simulink library "Lib_FileLogger"  (R2012b)
settings: Solver=ode45  StartTime=0.0  StopTime=10.0  RelTol=1e-3
undefined symbols (not defined in the file): macaddr, modelConstants
libraries: Lib_FileLogger x5, simulink x3, xpcethernetlib x2, xpcutilitieslib x1, dspswit3 x1, dspmtrx3 x1
settings Model: Creator=gilja  LastModifiedBy=nptl

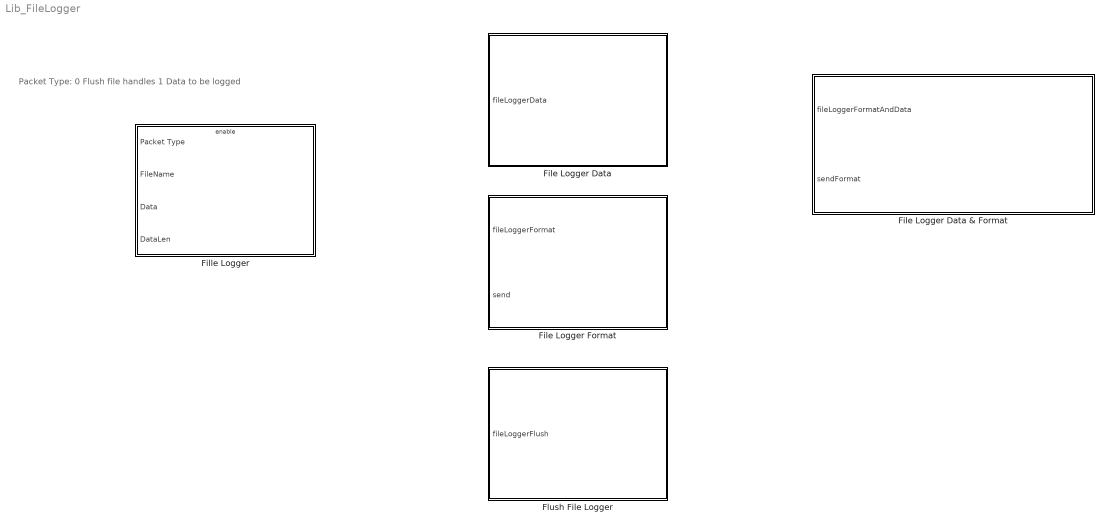
== system Lib_FileLogger ==
  note: Packet Type:
      | 0 Flush file handles
      | 1 Data to be logged
  File Logger Data : Subsystem
  File Logger Data & Format : Subsystem
  File Logger Format : Subsystem
  Fille Logger : Subsystem
  Flush File Logger : Subsystem

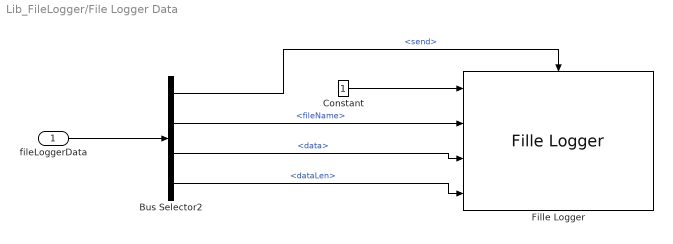
== system Lib_FileLogger/File Logger Data ==
  fileLoggerData : Inport  OutDataTypeStr=Bus: fileLoggerData
  Bus Selector2 : BusSelector  OutputSignals=send,fileName,data,dataLen
  Constant : Constant  OutDataTypeStr=boolean
  Fille Logger : Lib_FileLogger/Fille Logger
  wires:
  fileLoggerData/1 -> Bus Selector2/1
  Constant/1 -> Fille Logger/1
  Bus Selector2/1 -> Fille Logger/Enable  "<send>"
  Bus Selector2/4 -> Fille Logger/4  "<dataLen>"
  Bus Selector2/3 -> Fille Logger/3  "<data>"
  Bus Selector2/2 -> Fille Logger/2  "<fileName>"

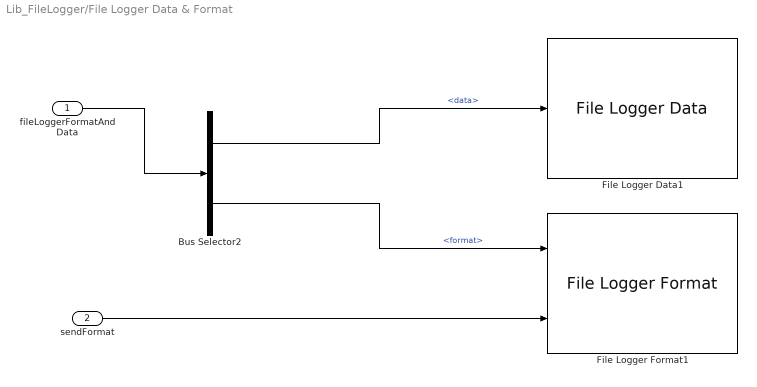
== system Lib_FileLogger/File Logger Data & Format ==
  fileLoggerFormatAndData : Inport  OutDataTypeStr=Bus: fileLoggerFormatAndData
  sendFormat : Inport  Port=2  OutDataTypeStr=boolean
  Bus Selector2 : BusSelector  OutputSignals=data,format
  File Logger Data1 : Lib_FileLogger/File Logger Data
  File Logger Format1 : Lib_FileLogger/File Logger Format
  wires:
  fileLoggerFormatAndData/1 -> Bus Selector2/1
  Bus Selector2/1 -> File Logger Data1/1  "<data>"
  Bus Selector2/2 -> File Logger Format1/1  "<format>"
  sendFormat/1 -> File Logger Format1/2

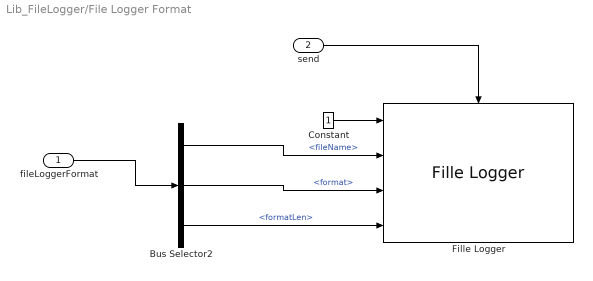
== system Lib_FileLogger/File Logger Format ==
  fileLoggerFormat : Inport  OutDataTypeStr=Bus: fileLoggerFormat
  send : Inport  Port=2  OutDataTypeStr=boolean
  Bus Selector2 : BusSelector  OutputSignals=fileName,format,formatLen
  Constant : Constant  OutDataTypeStr=boolean
  Fille Logger : Lib_FileLogger/Fille Logger
  wires:
  fileLoggerFormat/1 -> Bus Selector2/1
  send/1 -> Fille Logger/Enable
  Constant/1 -> Fille Logger/1
  Bus Selector2/3 -> Fille Logger/4  "<formatLen>"
  Bus Selector2/2 -> Fille Logger/3  "<format>"
  Bus Selector2/1 -> Fille Logger/2  "<fileName>"

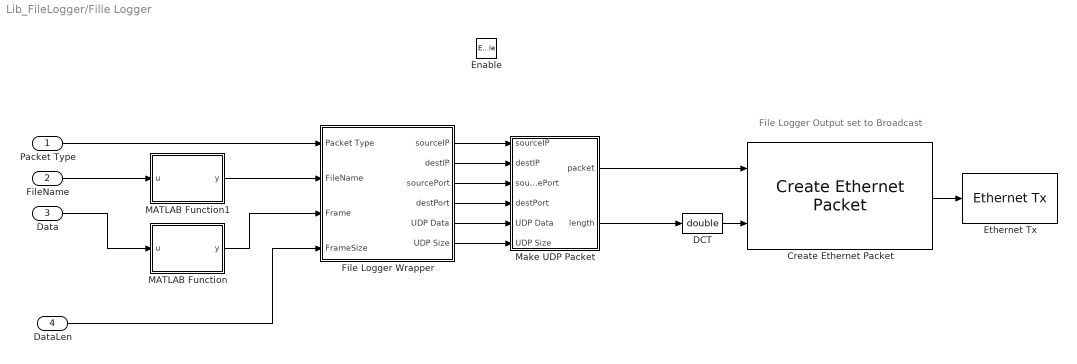
== system Lib_FileLogger/Fille Logger ==
  note: File Logger Output set to Broadcast
  Packet Type : Inport
  FileName : Inport  Port=2
  Data : Inport  Port=3
  DataLen : Inport  Port=4
  Enable : EnablePort
  "Create Ethernet Packet " : xpcethernetlib/Create Ethernet Packet   DstMac=macaddr('FF:FF:FF:FF:FF:FF')  EtherType=hex2dec('0800')
  DCT : DataTypeConversion  OutDataTypeStr=double
  "Ethernet Tx " : xpcethernetlib/Ethernet Tx   ID=2  SampleTime=-1
  File Logger Wrapper : Subsystem
  MATLAB Function : MATLAB Function  TreatAsAtomicUnit=on
  MATLAB Function1 : MATLAB Function  TreatAsAtomicUnit=on
  Make UDP Packet : Subsystem
  wires:
  FileName/1 -> MATLAB Function1/1(u)
  Data/1 -> MATLAB Function/1(u)
  File Logger Wrapper/1(sourceIP) -> Make UDP Packet/1(sourceIP)
  File Logger Wrapper/4(destPort) -> Make UDP Packet/4(destPort)
  Make UDP Packet/1(packet) -> "Create Ethernet Packet "/1
  "Create Ethernet Packet "/1 -> "Ethernet Tx "/1
  File Logger Wrapper/3(sourcePort) -> Make UDP Packet/3(sourcePort)
  Packet Type/1 -> File Logger Wrapper/1(Packet Type)
  MATLAB Function1/1(y) -> File Logger Wrapper/2(FileName)
  DCT/1 -> "Create Ethernet Packet "/2
  File Logger Wrapper/6(UDP Size) -> Make UDP Packet/6(UDP Size)
  Make UDP Packet/2(length) -> DCT/1
  DataLen/1 -> File Logger Wrapper/4(FrameSize)
  File Logger Wrapper/5(UDP Data) -> Make UDP Packet/5(UDP Data)
  File Logger Wrapper/2(destIP) -> Make UDP Packet/2(destIP)
  MATLAB Function/1(y) -> File Logger Wrapper/3(Frame)

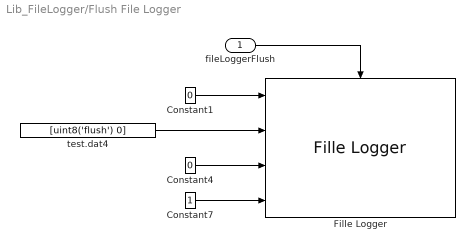
== system Lib_FileLogger/Flush File Logger ==
  fileLoggerFlush : Inport  OutDataTypeStr=boolean
  Constant1 : Constant  Value=0  OutDataTypeStr=boolean
  Constant4 : Constant  Value=0  OutDataTypeStr=boolean
  Constant7 : Constant  OutDataTypeStr=uint16
  Fille Logger : Lib_FileLogger/Fille Logger
  test.dat4 : Constant  Value=[uint8('flush') 0]  OutDataTypeStr=uint8
  wires:
  Constant4/1 -> Fille Logger/3
  fileLoggerFlush/1 -> Fille Logger/Enable
  Constant7/1 -> Fille Logger/4
  Constant1/1 -> Fille Logger/1
  test.dat4/1 -> Fille Logger/2

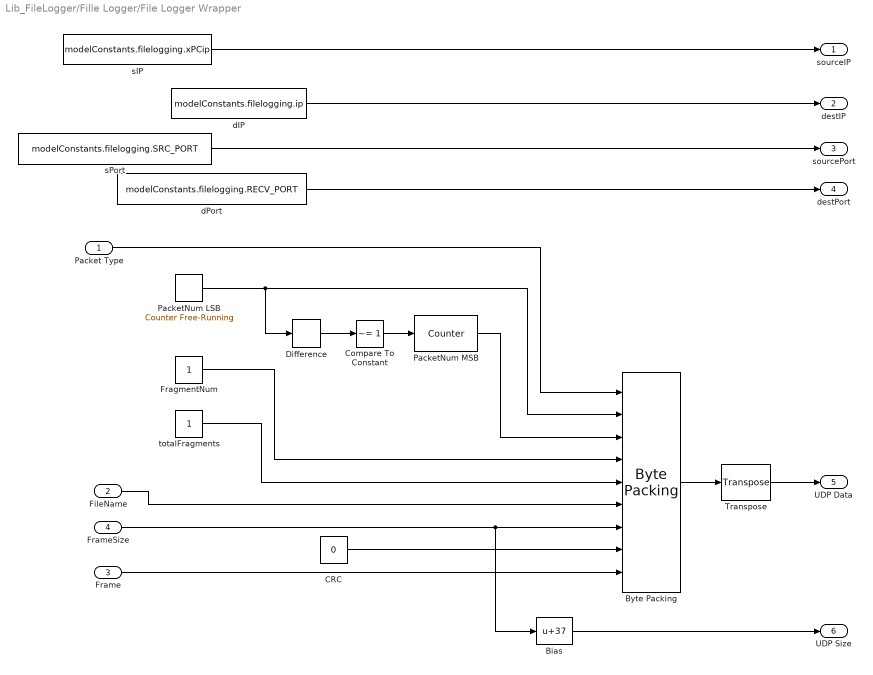
== system Lib_FileLogger/Fille Logger/File Logger Wrapper ==
  Packet Type : Inport
  FileName : Inport  Port=2
  Frame : Inport  Port=3
  FrameSize : Inport  Port=4
  Bias : Bias  Bias=37
  "Byte Packing " : xpcutilitieslib/Byte Packing   MaskPackedDataType=uint8  MaskUnpackedDataTypes={'boolean' 'uint32' 'uint32' 'uint8' 'uint8' 'uint8' 'uint16' 'uint32' 'uint8'}  MaskAlignment=1
  CRC : Constant  Value=0  OutDataTypeStr=uint32
  Compare To Constant : simulink/Logic and Bit Operations/Compare To Constant  relop=~=  const=1  OutDataTypeStr=uint8  ZeroCross=off
  Difference : simulink/Discrete/Difference  ICPrevInput=0  InputProcessing=Inherited  OutMin=[]  OutMax=[]  OutDataType=fixdt(1, 16)  OutScaling=2^-10  DoSatur=off
  FragmentNum : Constant  OutDataTypeStr=uint8
  PacketNum LSB : simulink/Sources/Counter Free-Running  NumBits=32  tsamp=-1
  PacketNum MSB : dspswit3/Counter  Direction=Up  CountEvent=Non-zero sample  CounterSize=32 bits  MaxCount=255  InitialCount=0  Output=Count  HitValue=32  ResetInput=off  SamplesPerFrame=1  Ts=1  CntDtype=uint32  HitDtype=Logical
  Transpose : dspmtrx3/Transpose  Hermitian=off  overflowFlag=off
  dIP : Constant  Value=modelConstants.filelogging.ip  OutDataTypeStr=uint8
  dPort : Constant  Value=modelConstants.filelogging.RECV_PORT  OutDataTypeStr=uint16
  sIP : Constant  Value=modelConstants.filelogging.xPCip  OutDataTypeStr=uint8
  sPort : Constant  Value=modelConstants.filelogging.SRC_PORT  OutDataTypeStr=uint16
  totalFragments : Constant  OutDataTypeStr=uint8
  sourceIP : Outport
  destIP : Outport  Port=2
  sourcePort : Outport  Port=3
  destPort : Outport  Port=4
  UDP Data : Outport  Port=5
  UDP Size : Outport  Port=6
  wires:
  Transpose/1 -> UDP Data/1
  "Byte Packing "/1 -> Transpose/1
  Frame/1 -> "Byte Packing "/9
  FrameSize/1 -> Bias/1, "Byte Packing "/7
  CRC/1 -> "Byte Packing "/8
  PacketNum MSB/1 -> "Byte Packing "/3
  Compare To Constant/1 -> PacketNum MSB/1
  Difference/1 -> Compare To Constant/1
  Packet Type/1 -> "Byte Packing "/1
  PacketNum LSB/1 -> "Byte Packing "/2, Difference/1
  FragmentNum/1 -> "Byte Packing "/4
  totalFragments/1 -> "Byte Packing "/5
  FileName/1 -> "Byte Packing "/6
  Bias/1 -> UDP Size/1
  dPort/1 -> destPort/1
  sPort/1 -> sourcePort/1
  dIP/1 -> destIP/1
  sIP/1 -> sourceIP/1

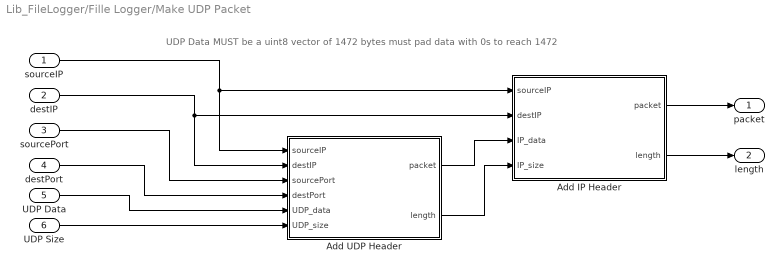
== system Lib_FileLogger/Fille Logger/Make UDP Packet ==
  note: UDP Data MUST be a uint8 vector of 1472 bytes
      | must pad data with 0s to reach 1472
  sourceIP : Inport
  destIP : Inport  Port=2
  sourcePort : Inport  Port=3
  destPort : Inport  Port=4
  UDP Data : Inport  Port=5
  UDP Size : Inport  Port=6
  Add IP Header : MATLAB Function  TreatAsAtomicUnit=on
  Add UDP Header : MATLAB Function  TreatAsAtomicUnit=on
  packet : Outport
  length : Outport  Port=2
  wires:
  UDP Size/1 -> Add UDP Header/6(UDP_size)
  Add IP Header/2(length) -> length/1
  Add IP Header/1(packet) -> packet/1
  UDP Data/1 -> Add UDP Header/5(UDP_data)
  destPort/1 -> Add UDP Header/4(destPort)
  sourcePort/1 -> Add UDP Header/3(sourcePort)
  destIP/1 -> Add IP Header/2(destIP), Add UDP Header/2(destIP)
  sourceIP/1 -> Add IP Header/1(sourceIP), Add UDP Header/1(sourceIP)
  Add UDP Header/1(packet) -> Add IP Header/3(IP_data)
  Add UDP Header/2(length) -> Add IP Header/4(IP_size)

== matlab function Lib_FileLogger/Fille Logger/MATLAB Function ==
  data: u input; y output
function y = padData(u)

z = uint8(zeros(1435, 1))';

z(1:length(u)) = u;

y = z';

== matlab function Lib_FileLogger/Fille Logger/MATLAB Function1 ==
  data: u input; y output
function y = padFileName(u)

z = uint8(zeros(20, 1));

z(1:length(u)) = u;

y = z';

== matlab function Lib_FileLogger/Fille Logger/Make UDP Packet/Add IP Header ==
  data: sourceIP input uint8 size=[1 4]; packet output uint8; destIP input uint8 size=[1 4]; IP_data input uint8; IP_size input uint16 size=[1 1]; length output uint16 size=[1 1]
function [packet, length] = makeIP(sourceIP, destIP, IP_data, IP_size)
% create IP packet

FFFF = uint16(hex2dec('FFFF'));

version_IHL = uint8(69); % IPv4 and IP header length of 5
ToS = uint8(0); % no QOS on network

length = IP_size + uint16(20); % hardcode header length to 5

length_BE = (typecast(length, 'uint8')); % change to big endian
length_BE = length_BE(end:-1:1);

% counter
persistent ID % identification
if isempty(ID)
    ID = uint16(0);
else
    ID = ID + 1;
end

ff = [ uint8(bin2dec('01000000')) 0 ]; % don't fragment packets

TTL = uint8(10); % ttl to 10 seconds/hops

protocol = uint8(hex2dec('11')); % UDP Protocol


header = [ version_IHL ToS length_BE typecast(ID, 'uint8') ff TTL protocol 0 0 sourceIP destIP];

% header(11:12) = typecast(bitcmp(uint16(sum( typecast(bitcmp(header), 'uint16') ))), 'uint8'); % checksum

checksum = FFFF - uint16(mod( uint32(sum( typecast(header, 'uint16') )), uint32(FFFF) ));
header(11:12) = typecast(checksum, 'uint8');

packet = [ header IP_data ];

== matlab function Lib_FileLogger/Fille Logger/Make UDP Packet/Add UDP Header ==
  data: sourceIP input uint8 size=[1 4]; packet output; destIP input uint8 size=[1 4]; sourcePort input uint16 size=[1 1]; destPort input uint16 size=[1 1]; UDP_data input uint8; UDP_size input uint16 size=[1 1]; length output uint16 size=[1 1]
function [packet, length] = makeUDP(sourceIP, destIP, sourcePort, destPort, UDP_data, UDP_size)
% create UDP packet

% sourceIP and destIP are 1x4 uint8 of the IP (in address order)
% sourcePort and destPort are uint16
% UDP_data is uint8 of 1xN packet data
% UDP_size is uint16 size of UDP_data
%
% NOTE: UDP_size MUST BE EVEN
FFFF = uint16(hex2dec('FFFF'));

protocol = uint8(hex2dec('11'));

length = UDP_size + uint16(8);

length_BE = (typecast(length, 'uint8')); % flip to big endian
length_BE = length_BE(end:-1:1);

sourcePort_BE = (typecast(sourcePort, 'uint8'));
sourcePort_BE = sourcePort_BE(end:-1:1);

destPort_BE   = (typecast(destPort,   'uint8'));
destPort_BE = destPort_BE(end:-1:1);

header = [sourcePort_BE destPort_BE length_BE uint8([0 0])];

pseudoHeader = [sourceIP destIP uint8(0) protocol length_BE];

% header(7:8) = typecast( bitcmp(uint16(sum( typecast(bitcmp([pseudoHeader header UDP_data]), 'uint16') ))), 'uint8');


checksum = FFFF - uint16(mod( uint32(sum( typecast([pseudoHeader header UDP_data], 'uint16') )), uint32(FFFF) ));
header(7:8) = typecast(checksum, 'uint8');

packet = [ header UDP_data ];
